simulink library "NMEA"  (R2024a)
settings: Solver=VariableStepAuto  StartTime=0.0  StopTime=10.0  RelTol=1e-3
libraries: $bdroot x44, simulink x21, simulink_extras x17, etargetslib x14
(part 2 of 4)

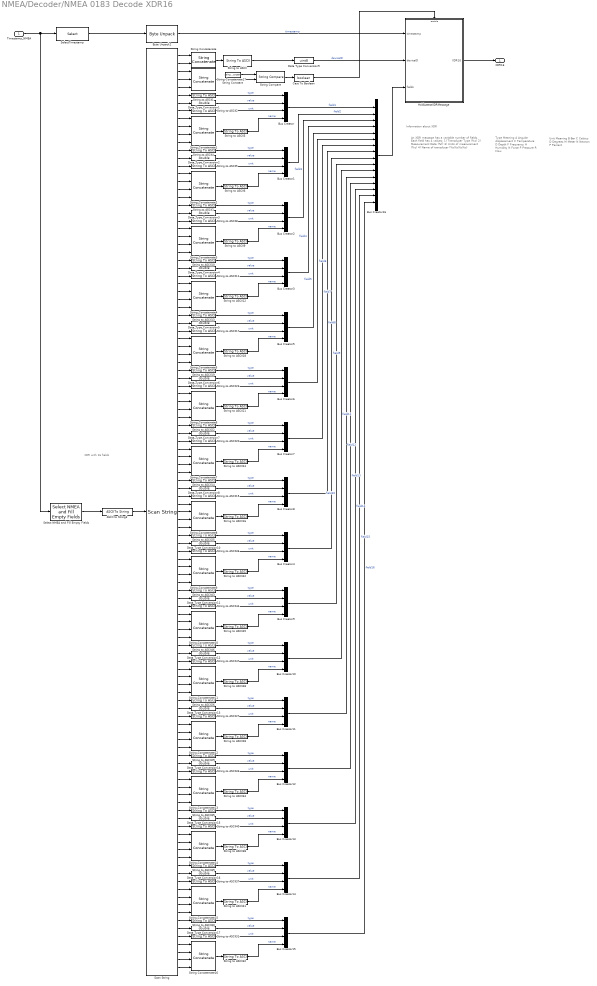
== system NMEA/Decoder/NMEA 0183 Decode XDR16 ==
  note: An XDR message has a variable number of fields.
      | Each field has 4 values:
      | 	1) Transducer Type (%c)
      | 	2) Measurement Data (%f)
      | 	3) Units of measurement (%c)
      | 	4) Name of transducer (%c%c%c%c)
  note: Type
      | Meaning
      |
      | A
      | Angular displacement
      |
      | C
      | Temperature
      |
      | D
      | Depth
      |
      | F
      | Frequency
      |
      | H
      | Humidity
      |
      | N
      | Force
      |
      | P
      | Pressure
      |
      | R
      | Flow
  note: Unit
      | Meaning
      |
      | B
      | Bar
      |
      | C
      | Celsius
      |
      | D
      | Degrees
      |
      | M
      | Meter
      |
      | N
      | Newton
      |
      | P
      | Percent
  note: Information about XDR
  note: XDR with 16 fields
  Timestamp_NMEA : Inport
  ASCII to String3 : ASCIIToString
  Bus Creator{,1..15} (16 alike) : BusCreator  Inputs=4
  Bus Creator16 : BusCreator  Inputs=16
  Byte Unpack2 : etargetslib/Byte Unpack  dimensions={1}  datatypes={'double'}  byteAlign=1
  Cast To Boolean : DataTypeConversion  OutDataTypeStr=boolean  SaturateOnIntegerOverflow=off  RndMeth=Floor
  Data Type Conversion{1..8,10..17} (16 alike) : DataTypeConversion  OutDataTypeStr=double  SaturateOnIntegerOverflow=off  RndMeth=Floor
  Data Type Conversion9 : DataTypeConversion  OutDataTypeStr=uint8  SaturateOnIntegerOverflow=off  RndMeth=Floor
  HoldLatestXDRMessage : Subsystem
  Scan String : ScanString  Format="\"$%c%c%c%c%c,%c,%lf,%c,%c%c%c%c,%c,%lf,%c,%c%c%c%c,%c,%lf,%c,%c%c%c%c,%c,%lf,%c,%c%c%c%c,%c,%lf,%c,%c%c%c%c,%c,%lf,%c,%c%c%c%c,%c,%lf,%c,%c%c%c%c,%c,%lf,%c,%c%c%c%c,%c,%lf,%c,%c%c%c%c,%c,%lf,%c,%c%c%c%c,%c,%lf,%c,%c%c%c%c,%c,%lf,%c,%c%c%c%c,%c,%lf,%c,%c%c%c%c,%c,%lf,%c,%c%c%c%c,%c,%lf,%c,%c%c%c%c,%c,%lf,%c,%c%c%c%c\""
  Select NMEA and Fill Empty Fields : $bdroot/Details/Select NMEA and Fill Empty Fields
  SelectTimestamp : Selector  IndexOptions=Index vector (dialog)  Indices=1:8  OutputSizes=1
  String Compare : StringCompare
  String Concatenate : StringConcatenate
  String Concatenate{1..16} (16 alike) : StringConcatenate  Inputs=4
  String Concatenate17 : StringConcatenate  Inputs=3
  String Constant : StringConstant  String="\"XDR\""
  String to ASCII : StringToASCII
  String to ASCII{1..2,4..5,7..8,10..11,13..15,17,19..20,22..23,25..27,29..31,33,35..37,39..40,43..44,46..47} (32 alike) : StringToASCII  OutputVectorSize=1
  String to ASCII{3,6,9,12,16,18,21,24,28,32,34,38,41..42,45,48} (16 alike) : StringToASCII  OutputVectorSize=4
  XDR16 : Outport
  wires:
  String to ASCII7/1 -> Bus Creator2/1  "type"
  Data Type Conversion3/1 -> Bus Creator2/2  "value"
  String to ASCII8/1 -> Bus Creator2/3  "unit"
  String Concatenate3/1 -> String to ASCII9/1
  String to ASCII9/1 -> Bus Creator2/4  "name"
  String to ASCII12/1 -> Bus Creator3/4  "name"
  String Concatenate4/1 -> String to ASCII12/1
  String to ASCII11/1 -> Bus Creator3/3  "unit"
  Data Type Conversion4/1 -> Bus Creator3/2  "value"
  String to ASCII10/1 -> Bus Creator3/1  "type"
  String to ASCII4/1 -> Bus Creator1/1  "type"
  Data Type Conversion2/1 -> Bus Creator1/2  "value"
  String to ASCII5/1 -> Bus Creator1/3  "unit"
  String Concatenate2/1 -> String to ASCII6/1
  String to ASCII6/1 -> Bus Creator1/4  "name"
  String to ASCII3/1 -> Bus Creator/4  "name"
  String Concatenate1/1 -> String to ASCII3/1
  String to ASCII2/1 -> Bus Creator/3  "unit"
  Data Type Conversion1/1 -> Bus Creator/2  "value"
  String to ASCII1/1 -> Bus Creator/1  "type"
  Scan String/1 -> String Concatenate/1
  Select NMEA and Fill Empty Fields/1 -> ASCII to String3/1
  SelectTimestamp/1 -> Byte Unpack2/1
  Timestamp_NMEA/1 -> Select NMEA and Fill Empty Fields/1, SelectTimestamp/1
  ASCII to String3/1 -> Scan String/1
  Scan String/2 -> String Concatenate/2
  String to ASCII13/1 -> Bus Creator5/1  "type"
  Data Type Conversion5/1 -> Bus Creator5/2  "value"
  String to ASCII17/1 -> Bus Creator5/3  "unit"
  String Concatenate5/1 -> String to ASCII18/1
  String to ASCII18/1 -> Bus Creator5/4  "name"
  String to ASCII21/1 -> Bus Creator6/4  "name"
  String Concatenate6/1 -> String to ASCII21/1
  String to ASCII23/1 -> Bus Creator6/3  "unit"
  Data Type Conversion6/1 -> Bus Creator6/2  "value"
  String to ASCII19/1 -> Bus Creator6/1  "type"
  String to ASCII14/1 -> Bus Creator8/1  "type"
  Data Type Conversion8/1 -> Bus Creator8/2  "value"
  String to ASCII15/1 -> Bus Creator8/3  "unit"
  String Concatenate8/1 -> String to ASCII16/1
  String to ASCII16/1 -> Bus Creator8/4  "name"
  String to ASCII24/1 -> Bus Creator7/4  "name"
  String Concatenate7/1 -> String to ASCII24/1
  String to ASCII20/1 -> Bus Creator7/3  "unit"
  Data Type Conversion7/1 -> Bus Creator7/2  "value"
  String to ASCII22/1 -> Bus Creator7/1  "type"
  String to ASCII/1 -> Data Type Conversion9/1
  String Concatenate/1 -> String to ASCII/1
  String to ASCII39/1 -> Bus Creator14/1  "type"
  Data Type Conversion16/1 -> Bus Creator14/2  "value"
  String to ASCII37/1 -> Bus Creator14/3  "unit"
  String Concatenate15/1 -> String to ASCII41/1
  String to ASCII41/1 -> Bus Creator14/4  "name"
  String to ASCII32/1 -> Bus Creator15/4  "name"
  String Concatenate16/1 -> String to ASCII32/1
  String to ASCII31/1 -> Bus Creator15/3  "unit"
  Data Type Conversion17/1 -> Bus Creator15/2  "value"
  String to ASCII30/1 -> Bus Creator15/1  "type"
  String to ASCII35/1 -> Bus Creator13/1  "type"
  Data Type Conversion15/1 -> Bus Creator13/2  "value"
  String to ASCII40/1 -> Bus Creator13/3  "unit"
  String Concatenate14/1 -> String to ASCII38/1
  String to ASCII38/1 -> Bus Creator13/4  "name"
  String to ASCII34/1 -> Bus Creator12/4  "name"
  String Concatenate13/1 -> String to ASCII34/1
  String to ASCII33/1 -> Bus Creator12/3  "unit"
  Data Type Conversion14/1 -> Bus Creator12/2  "value"
  String to ASCII29/1 -> Bus Creator12/1  "type"
  String to ASCII25/1 -> Bus Creator4/1  "type"
  Data Type Conversion10/1 -> Bus Creator4/2  "value"
  String to ASCII36/1 -> Bus Creator4/3  "unit"
  String Concatenate9/1 -> String to ASCII42/1
  String to ASCII42/1 -> Bus Creator4/4  "name"
  String to ASCII45/1 -> Bus Creator9/4  "name"
  String Concatenate10/1 -> String to ASCII45/1
  String to ASCII44/1 -> Bus Creator9/3  "unit"
  Data Type Conversion11/1 -> Bus Creator9/2  "value"
  String to ASCII43/1 -> Bus Creator9/1  "type"
  String to ASCII26/1 -> Bus Creator11/1  "type"
  Data Type Conversion13/1 -> Bus Creator11/2  "value"
  String to ASCII27/1 -> Bus Creator11/3  "unit"
  String Concatenate12/1 -> String to ASCII28/1
  String to ASCII28/1 -> Bus Creator11/4  "name"
  String to ASCII48/1 -> Bus Creator10/4  "name"
  String Concatenate11/1 -> String to ASCII48/1
  String to ASCII47/1 -> Bus Creator10/3  "unit"
  Data Type Conversion12/1 -> Bus Creator10/2  "value"
  String to ASCII46/1 -> Bus Creator10/1  "type"
  Scan String/3 -> String Concatenate17/1
  Scan String/4 -> String Concatenate17/2
  Scan String/5 -> String Concatenate17/3
  String Concatenate17/1 -> String Compare/2
  String Constant/1 -> String Compare/1
  String Compare/1 -> Cast To Boolean/1
  Scan String/6 -> String to ASCII1/1
  Scan String/7 -> Data Type Conversion1/1
  Scan String/8 -> String to ASCII2/1
  Scan String/9 -> String Concatenate1/1
  Scan String/10 -> String Concatenate1/2
  Scan String/11 -> String Concatenate1/3
  Scan String/12 -> String Concatenate1/4
  Scan String/13 -> String to ASCII4/1
  Scan String/14 -> Data Type Conversion2/1
  Scan String/15 -> String to ASCII5/1
  Scan String/16 -> String Concatenate2/1
  Scan String/17 -> String Concatenate2/2
  Scan String/18 -> String Concatenate2/3
  Scan String/19 -> String Concatenate2/4
  Scan String/20 -> String to ASCII7/1
  Scan String/21 -> Data Type Conversion3/1
  Scan String/22 -> String to ASCII8/1
  Scan String/23 -> String Concatenate3/1
  Scan String/24 -> String Concatenate3/2
  Scan String/25 -> String Concatenate3/3
  Scan String/26 -> String Concatenate3/4
  Scan String/27 -> String to ASCII10/1
  Scan String/28 -> Data Type Conversion4/1
  Scan String/29 -> String to ASCII11/1
  Scan String/30 -> String Concatenate4/1
  Scan String/31 -> String Concatenate4/2
  Scan String/32 -> String Concatenate4/3
  Scan String/33 -> String Concatenate4/4
  Scan String/34 -> String to ASCII13/1
  Scan String/35 -> Data Type Conversion5/1
  Scan String/36 -> String to ASCII17/1
  Scan String/37 -> String Concatenate5/1
  Scan String/38 -> String Concatenate5/2
  Scan String/39 -> String Concatenate5/3
  Scan String/40 -> String Concatenate5/4
  Scan String/41 -> String to ASCII19/1
  Scan String/42 -> Data Type Conversion6/1
  Scan String/43 -> String to ASCII23/1
  Scan String/44 -> String Concatenate6/1
  Scan String/45 -> String Concatenate6/2
  Scan String/46 -> String Concatenate6/3
  Scan String/47 -> String Concatenate6/4
  Scan String/48 -> String to ASCII22/1
  Scan String/49 -> Data Type Conversion7/1
  Scan String/50 -> String to ASCII20/1
  Scan String/51 -> String Concatenate7/1
  Scan String/52 -> String Concatenate7/2
  Scan String/53 -> String Concatenate7/3
  Scan String/54 -> String Concatenate7/4
  Scan String/55 -> String to ASCII14/1
  Scan String/56 -> Data Type Conversion8/1
  Scan String/57 -> String to ASCII15/1
  Scan String/58 -> String Concatenate8/1
  Scan String/59 -> String Concatenate8/2
  Scan String/60 -> String Concatenate8/3
  Scan String/61 -> String Concatenate8/4
  Scan String/62 -> String to ASCII25/1
  Scan String/63 -> Data Type Conversion10/1
  Scan String/64 -> String to ASCII36/1
  Scan String/65 -> String Concatenate9/1
  Scan String/66 -> String Concatenate9/2
  Scan String/67 -> String Concatenate9/3
  Scan String/68 -> String Concatenate9/4
  Scan String/69 -> String to ASCII43/1
  Scan String/70 -> Data Type Conversion11/1
  Scan String/71 -> String to ASCII44/1
  Scan String/72 -> String Concatenate10/1
  Scan String/73 -> String Concatenate10/2
  Scan String/74 -> String Concatenate10/3
  Scan String/75 -> String Concatenate10/4
  Scan String/76 -> String to ASCII46/1
  Scan String/77 -> Data Type Conversion12/1
  Scan String/78 -> String to ASCII47/1
  Scan String/79 -> String Concatenate11/1
  Scan String/80 -> String Concatenate11/2
  Scan String/81 -> String Concatenate11/3
  Scan String/82 -> String Concatenate11/4
  Scan String/83 -> String to ASCII26/1
  Scan String/84 -> Data Type Conversion13/1
  Scan String/85 -> String to ASCII27/1
  Scan String/86 -> String Concatenate12/1
  Scan String/87 -> String Concatenate12/2
  Scan String/88 -> String Concatenate12/3
  Scan String/89 -> String Concatenate12/4
  Scan String/90 -> String to ASCII29/1
  Scan String/91 -> Data Type Conversion14/1
  Scan String/92 -> String to ASCII33/1
  Scan String/93 -> String Concatenate13/1
  Scan String/94 -> String Concatenate13/2
  Scan String/95 -> String Concatenate13/3
  Scan String/96 -> String Concatenate13/4
  Scan String/97 -> String to ASCII35/1
  Scan String/98 -> Data Type Conversion15/1
  Scan String/99 -> String to ASCII40/1
  Scan String/100 -> String Concatenate14/1
  Scan String/101 -> String Concatenate14/2
  Scan String/102 -> String Concatenate14/3
  Scan String/103 -> String Concatenate14/4
  Scan String/104 -> String to ASCII39/1
  Scan String/105 -> Data Type Conversion16/1
  Scan String/106 -> String to ASCII37/1
  Scan String/107 -> String Concatenate15/1
  Scan String/108 -> String Concatenate15/2
  Scan String/109 -> String Concatenate15/3
  Scan String/110 -> String Concatenate15/4
  Scan String/111 -> String to ASCII30/1
  Scan String/112 -> Data Type Conversion17/1
  Scan String/113 -> String to ASCII31/1
  Scan String/114 -> String Concatenate16/1
  Scan String/115 -> String Concatenate16/2
  Scan String/116 -> String Concatenate16/3
  Scan String/117 -> String Concatenate16/4
  Bus Creator9/1 -> Bus Creator16/10  "field10"
  Bus Creator4/1 -> Bus Creator16/9  "field9"
  Bus Creator10/1 -> Bus Creator16/11  "field11"
  Bus Creator8/1 -> Bus Creator16/8  "field8"
  Bus Creator11/1 -> Bus Creator16/12  "field12"
  Bus Creator7/1 -> Bus Creator16/7  "field7"
  Bus Creator12/1 -> Bus Creator16/13  "field13"
  Bus Creator6/1 -> Bus Creator16/6  "field6"
  Bus Creator13/1 -> Bus Creator16/14  "field14"
  Bus Creator5/1 -> Bus Creator16/5  "field5"
  Bus Creator14/1 -> Bus Creator16/15  "field15"
  Bus Creator3/1 -> Bus Creator16/4  "field4"
  Bus Creator15/1 -> Bus Creator16/16  "field16"
  Bus Creator2/1 -> Bus Creator16/3  "field3"
  Bus Creator1/1 -> Bus Creator16/2  "field2"
  Bus Creator/1 -> Bus Creator16/1  "field1"
  Bus Creator16/1 -> HoldLatestXDRMessage/3(fields)
  Data Type Conversion9/1 -> HoldLatestXDRMessage/2(deviceID)  "deviceID"
  Byte Unpack2/1 -> HoldLatestXDRMessage/1(timestamp)  "timestamp"
  Cast To Boolean/1 -> HoldLatestXDRMessage/Enable
  HoldLatestXDRMessage/1(XDR16) -> XDR16/1

== system NMEA/Decoder/NMEA 0183 Decode ZDA ==
  Timestamp_NMEA : Inport
  ASCII to String3 : ASCIIToString
  Byte Unpack2 : etargetslib/Byte Unpack  dimensions={1}  datatypes={'double'}  byteAlign=1
  Compare To Constant : simulink/Logic and Bit Operations/Compare To Constant  relop===  const=uint8(42)  OutDataTypeStr=boolean
  DecodeMessage : Subsystem  TreatAsAtomicUnit=on
  Scan String : ScanString  Format="\"$%c%cZDA,%02u%02u%lf,%02u,%02u,%u,%02u,%02u%c\""
  Select NMEA and Fill Empty Fields : $bdroot/Details/Select NMEA and Fill Empty Fields
  SelectTimestamp : Selector  IndexOptions=Index vector (dialog)  Indices=1:8  OutputSizes=1
  String Concatenate : StringConcatenate
  String to ASCII : StringToASCII  OutputVectorSize=1
  ZDA : Outport
  wires:
  Compare To Constant/1 -> DecodeMessage/Enable
  Scan String/2 -> String Concatenate/2
  String Concatenate/1 -> DecodeMessage/2(strID)
  ASCII to String3/1 -> Scan String/1
  Timestamp_NMEA/1 -> Select NMEA and Fill Empty Fields/1, SelectTimestamp/1
  DecodeMessage/1(ZDA) -> ZDA/1
  Byte Unpack2/1 -> DecodeMessage/1(timestamp)  "timestamp"
  Scan String/11 -> String to ASCII/1
  SelectTimestamp/1 -> Byte Unpack2/1
  String to ASCII/1 -> Compare To Constant/1
  Select NMEA and Fill Empty Fields/1 -> ASCII to String3/1
  Scan String/1 -> String Concatenate/1
  Scan String/3 -> DecodeMessage/3(utcHour)
  Scan String/4 -> DecodeMessage/4(utcMinute)
  Scan String/5 -> DecodeMessage/5(utcSecond)
  Scan String/6 -> DecodeMessage/6(utcDay)
  Scan String/7 -> DecodeMessage/7(utcMonth)
  Scan String/8 -> DecodeMessage/8(utcYear)
  Scan String/9 -> DecodeMessage/9(localTimeZoneOffsetFromGMTHour)
  Scan String/10 -> DecodeMessage/10(localTimeZoneOffsetFromGMTMinute)

== system NMEA/Details/Append CR LF ==
  bytesIn : Inport  OutDataTypeStr=uint8
  lengthIn : Inport  Port=2  OutDataTypeStr=uint32  PortDimensions=1
  Assignment : Assignment  DiagnosticForDimensions=Warning  IndexOptions=Index vector (port)  Indices=1  OutputSizes=1
  Bias : Bias  Bias=int32(1)  SaturateOnIntegerOverflow=off
  Bias1 : Bias  Bias=int32(2)  SaturateOnIntegerOverflow=off
  Bias2 : Bias  Bias=uint32(2)  SaturateOnIntegerOverflow=off
  Compare To Constant : simulink/Logic and Bit Operations/Compare To Constant  relop=>  const=int32(1)  OutDataTypeStr=boolean
  Constant : Constant  Value=int32(1)
  Constant81 : Constant  Value=int32(1)
  Constant82 : Constant  Value=uint8(13)
  Constant83 : Constant  Value=uint8(10)
  Data Type Conversion : DataTypeConversion  OutDataTypeStr=int32  SaturateOnIntegerOverflow=off  RndMeth=Floor
  Mux{,1..3} (4 alike) : Mux  Inputs=2
  Selector : Selector  IndexOptions=Index vector (dialog)  Indices=1  OutputSizes=1
  Selector1 : Selector  IndexOptions=Index vector (dialog)  Indices=2  OutputSizes=1
  Sum : Sum  Inputs=|+-
  Switch : Switch  Criteria=u2 > Threshold  SaturateOnIntegerOverflow=off  InputSameDT=off
  Switch1 : Switch  Criteria=u2 > Threshold  SaturateOnIntegerOverflow=off  InputSameDT=off
  Switch2 : Switch  Criteria=u2 > Threshold  SaturateOnIntegerOverflow=off  InputSameDT=off
  Width : Width  DataType=int32
  bytesOut : Outport  OutDataTypeStr=uint8
  lengthOut : Outport  Port=2  OutDataTypeStr=uint32
  wires:
  Bias1/1 -> Mux/2
  Width/1 -> Sum/1
  Bias2/1 -> Switch2/1
  Constant/1 -> Mux1/1
  Compare To Constant/1 -> Switch2/2, Switch/2, Switch1/2
  Bias/1 -> Mux/1
  Mux3/1 -> Switch1/3
  lengthIn/1 -> Switch2/3, Bias2/1, Data Type Conversion/1
  Data Type Conversion/1 -> Bias1/1, Bias/1, Sum/2
  Mux/1 -> Switch/1
  bytesIn/1 -> Assignment/1, Selector1/1, Selector/1, Width/1
  Sum/1 -> Compare To Constant/1
  Mux2/1 -> Switch1/1
  Constant81/1 -> Mux1/2
  Constant82/1 -> Mux2/1
  Switch1/1 -> Assignment/2
  Switch/1 -> Assignment/3
  Mux1/1 -> Switch/3
  Selector/1 -> Mux3/1
  Selector1/1 -> Mux3/2
  Constant83/1 -> Mux2/2
  Assignment/1 -> bytesOut/1
  Switch2/1 -> lengthOut/1

== system NMEA/Details/Ensure Positive Angle ==
  x : Inport  OutDataTypeStr=double  Unit=rad
  Positive Angle : MATLAB Function  TreatAsAtomicUnit=on
  y : Outport  OutDataTypeStr=double  Unit=rad
  wires:
  Positive Angle/1(y) -> y/1
  x/1 -> Positive Angle/1(x)

== system NMEA/Details/Ensure Symmetrical Angle ==
  x : Inport  OutDataTypeStr=double  Unit=rad
  Symmetrical Angle : MATLAB Function  TreatAsAtomicUnit=on
  y : Outport  OutDataTypeStr=double  Unit=rad
  wires:
  x/1 -> Symmetrical Angle/1(x)
  Symmetrical Angle/1(y) -> y/1

== system NMEA/Details/NMEA Checksum Message ==
  note: Add checksum (output buffer size: 128)
  note: NMEA String including $ and *
  nmeaString : Inport
  MATLAB Function : MATLAB Function  TreatAsAtomicUnit=on
  bytes : Outport  OutDataTypeStr=uint8
  length : Outport  Port=2  OutDataTypeStr=uint32  PortDimensions=1
  wires:
  MATLAB Function/2(len) -> length/1
  MATLAB Function/1(bytes) -> bytes/1
  nmeaString/1 -> MATLAB Function/1(nmeaData)

== system NMEA/Details/NMEA Checksum Test ==
  bytes : Inport  OutDataTypeStr=uint8
  length : Inport  Port=2  OutDataTypeStr=uint32  PortDimensions=1
  MATLAB Function : MATLAB Function  TreatAsAtomicUnit=on
  isCorrect : Outport  OutDataTypeStr=boolean  PortDimensions=1
  wires:
  MATLAB Function/1(isCorrect) -> isCorrect/1
  bytes/1 -> MATLAB Function/1(bytes)
  length/1 -> MATLAB Function/2(len)

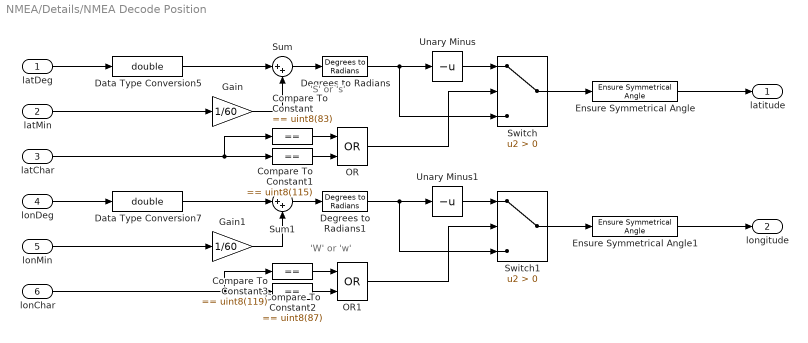
== system NMEA/Details/NMEA Decode Position ==
  note: 'S' or 's'
  note: 'W' or 'w'
  latDeg : Inport  OutDataTypeStr=uint32  Unit=deg  PortDimensions=1
  latMin : Inport  Port=2  OutDataTypeStr=double  Unit=min  PortDimensions=1
  latChar : Inport  Port=3  OutDataTypeStr=uint8  PortDimensions=1
  lonDeg : Inport  Port=4  OutDataTypeStr=uint32  Unit=deg  PortDimensions=1
  lonMin : Inport  Port=5  OutDataTypeStr=double  Unit=min  PortDimensions=1
  lonChar : Inport  Port=6  OutDataTypeStr=uint8  PortDimensions=1
  Compare To Constant : simulink/Logic and Bit Operations/Compare To Constant  relop===  const=uint8(83)  OutDataTypeStr=boolean
  Compare To Constant1 : simulink/Logic and Bit Operations/Compare To Constant  relop===  const=uint8(115)  OutDataTypeStr=boolean
  Compare To Constant2 : simulink/Logic and Bit Operations/Compare To Constant  relop===  const=uint8(87)  OutDataTypeStr=boolean
  Compare To Constant3 : simulink/Logic and Bit Operations/Compare To Constant  relop===  const=uint8(119)  OutDataTypeStr=boolean
  Data Type Conversion5 : DataTypeConversion  OutDataTypeStr=double  SaturateOnIntegerOverflow=off  RndMeth=Floor
  Data Type Conversion7 : DataTypeConversion  OutDataTypeStr=double  SaturateOnIntegerOverflow=off  RndMeth=Floor
  Degrees to Radians : simulink_extras/Transformations/Degrees to Radians
  Degrees to Radians1 : simulink_extras/Transformations/Degrees to Radians
  Ensure Symmetrical Angle : $bdroot/Details/Ensure Symmetrical Angle
  Ensure Symmetrical Angle1 : $bdroot/Details/Ensure Symmetrical Angle
  Gain : Gain  Gain=1/60
  Gain1 : Gain  Gain=1/60
  OR : Logic  Operator=OR  AllPortsSameDT=off  OutDataTypeStr=boolean
  OR1 : Logic  Operator=OR  AllPortsSameDT=off  OutDataTypeStr=boolean
  Sum : Sum  Inputs=|++
  Sum1 : Sum  Inputs=|++
  Switch : Switch  Criteria=u2 > Threshold  SaturateOnIntegerOverflow=off  InputSameDT=off
  Switch1 : Switch  Criteria=u2 > Threshold  SaturateOnIntegerOverflow=off  InputSameDT=off
  Unary Minus : UnaryMinus
  Unary Minus1 : UnaryMinus
  latitude : Outport  OutDataTypeStr=double  Unit=rad  PortDimensions=1
  longitude : Outport  Port=2  OutDataTypeStr=double  Unit=rad  PortDimensions=1
  wires:
  Data Type Conversion5/1 -> Sum/1
  Switch1/1 -> Ensure Symmetrical Angle1/1
  latDeg/1 -> Data Type Conversion5/1
  lonChar/1 -> Compare To Constant3/1, Compare To Constant2/1
  latMin/1 -> Gain/1
  Data Type Conversion7/1 -> Sum1/1
  Gain/1 -> Sum/2
  Compare To Constant/1 -> OR/1
  Unary Minus1/1 -> Switch1/1
  Sum/1 -> Degrees to Radians/1
  lonMin/1 -> Gain1/1
  Compare To Constant3/1 -> OR1/2
  latChar/1 -> Compare To Constant/1, Compare To Constant1/1
  OR/1 -> Switch/2
  Compare To Constant1/1 -> OR/2
  Unary Minus/1 -> Switch/1
  OR1/1 -> Switch1/2
  Gain1/1 -> Sum1/2
  Degrees to Radians/1 -> Switch/3, Unary Minus/1
  Sum1/1 -> Degrees to Radians1/1
  Degrees to Radians1/1 -> Unary Minus1/1, Switch1/3
  lonDeg/1 -> Data Type Conversion7/1
  Switch/1 -> Ensure Symmetrical Angle/1
  Compare To Constant2/1 -> OR1/1
  Ensure Symmetrical Angle/1 -> latitude/1
  Ensure Symmetrical Angle1/1 -> longitude/1

== system NMEA/Details/NMEA Encode Position ==
  lat : Inport  OutDataTypeStr=double  Unit=rad  PortDimensions=1
  lon : Inport  Port=2  OutDataTypeStr=double  Unit=rad  PortDimensions=1
  EncodePosition : MATLAB Function  TreatAsAtomicUnit=on
  latDeg : Outport  OutDataTypeStr=uint32  Unit=deg  PortDimensions=1
  latMin : Outport  Port=2  OutDataTypeStr=double  Unit=min  PortDimensions=1
  latChar : Outport  Port=3  OutDataTypeStr=uint8  PortDimensions=1
  lonDeg : Outport  Port=4  OutDataTypeStr=uint32  Unit=deg  PortDimensions=1
  lonMin : Outport  Port=5  OutDataTypeStr=double  Unit=min  PortDimensions=1
  lonChar : Outport  Port=6  OutDataTypeStr=uint8  PortDimensions=1
  wires:
  EncodePosition/2(latMin) -> latMin/1
  lat/1 -> EncodePosition/1(lat)
  lon/1 -> EncodePosition/2(lon)
  EncodePosition/3(latChar) -> latChar/1
  EncodePosition/4(lonDeg) -> lonDeg/1
  EncodePosition/1(latDeg) -> latDeg/1
  EncodePosition/6(lonChar) -> lonChar/1
  EncodePosition/5(lonMin) -> lonMin/1

== system NMEA/Details/NMEA Fill Empty Fields ==
  bytesIn : Inport  OutDataTypeStr=uint8
  lengthIn : Inport  Port=2  OutDataTypeStr=uint32  PortDimensions=1
  MATLAB Function : MATLAB Function  TreatAsAtomicUnit=on
  bytesOut : Outport  OutDataTypeStr=uint8
  lengthOut : Outport  Port=2  OutDataTypeStr=uint32  PortDimensions=1
  wires:
  MATLAB Function/1(bytesOut) -> bytesOut/1
  lengthIn/1 -> MATLAB Function/2(lengthIn)
  MATLAB Function/2(lengthOut) -> lengthOut/1
  bytesIn/1 -> MATLAB Function/1(bytesIn)

== system NMEA/Details/NMEA XDR16 Get Value Of Transducer ==
  note: Unit
      | Meaning
      |
      | B
      | Bar
      |
      | C
      | Celsius
      |
      | D
      | Degrees
      |
      | M
      | Meter
      |
      | N
      | Newton
      |
      | P
      | Percent
  note: Type
      | Meaning
      |
      | A
      | Angular displacement
      |
      | C
      | Temperature
      |
      | D
      | Depth
      |
      | F
      | Frequency
      |
      | H
      | Humidity
      |
      | N
      | Force
      |
      | P
      | Pressure
      |
      | R
      | Flow
  note: Information about XDR
  note: An XDR message has a variable number of fields.
      | Each field has 4 values:
      | 	1) Transducer Type (%c)
      | 	2) Measurement Data (%f)
      | 	3) Units of measurement (%c)
      | 	4) Name of transducer (%c%c%c%c)
  transducerName : Inport  OutDataTypeStr=uint8  PortDimensions=4
  XDR16 : Inport  Port=2
  Bus Selector1 : BusSelector  OutputSignals=types,values,units,names
  MATLAB Function : MATLAB Function  TreatAsAtomicUnit=on
  found : Outport  OutDataTypeStr=boolean  PortDimensions=1
  value : Outport  Port=2  OutDataTypeStr=double  PortDimensions=1
  wires:
  MATLAB Function/1(value) -> value/1
  Bus Selector1/4 -> MATLAB Function/5(namesXDR)  "<names>"
  XDR16/1 -> Bus Selector1/1
  Bus Selector1/1 -> MATLAB Function/2(typesXDR)  "<types>"
  Bus Selector1/2 -> MATLAB Function/3(valuesXDR)  "<values>"
  transducerName/1 -> MATLAB Function/1(transducerName)
  Bus Selector1/3 -> MATLAB Function/4(unitsXDR)  "<units>"
  MATLAB Function/2(found) -> found/1

== system NMEA/Details/Select NMEA and Fill Empty Fields ==
  Timestamp_NMEA : Inport
  SelectMessageAndFillEmptyFields : MATLAB Function  TreatAsAtomicUnit=on
  ASCII : Outport
  wires:
  Timestamp_NMEA/1 -> SelectMessageAndFillEmptyFields/1(u)
  SelectMessageAndFillEmptyFields/1(y) -> ASCII/1

== system NMEA/Encoder/NMEA 0183 Encode ALR ==
  note: Add checksum (output buffer size: 128)
  note: NMEA String including $ and *
  deviceID : Inport  OutDataTypeStr=uint8  PortDimensions=2
  utcHour : Inport  Port=2  OutDataTypeStr=uint32  PortDimensions=1
  utcMinute : Inport  Port=3  OutDataTypeStr=uint32  PortDimensions=1
  utcSecond : Inport  Port=4  OutDataTypeStr=double  Unit=s  PortDimensions=1
  alarmID1 : Inport  Port=5  OutDataTypeStr=uint32  PortDimensions=1
  alarmID2 : Inport  Port=6  OutDataTypeStr=uint32  PortDimensions=1
  alarmID3 : Inport  Port=7  OutDataTypeStr=uint32  PortDimensions=1
  alarmCondition : Inport  Port=8  OutDataTypeStr=uint8  PortDimensions=1
  alarmAcknowledge : Inport  Port=9  OutDataTypeStr=uint8  PortDimensions=1
  ASCII to String : ASCIIToString
  ASCII to String1 : ASCIIToString
  ASCII to String2 : ASCIIToString
  Compose String : ComposeString  Format="\"$%sALR,%02u%02u%05.2f,%u%u%u,%s,%s,*\""
  NMEA Checksum Message : $bdroot/Details/NMEA Checksum Message
  Saturation : Saturate  UpperLimit=uint32(9)  LowerLimit=uint32(0)
  Saturation1 : Saturate  UpperLimit=uint32(9)  LowerLimit=uint32(0)
  Saturation2 : Saturate  UpperLimit=uint32(9)  LowerLimit=uint32(0)
  bytes : Outport  OutDataTypeStr=uint8
  length : Outport  Port=2  OutDataTypeStr=uint32  PortDimensions=1
  wires:
  NMEA Checksum Message/1 -> bytes/1
  NMEA Checksum Message/2 -> length/1
  deviceID/1 -> ASCII to String/1
  ASCII to String/1 -> Compose String/1
  Compose String/1 -> NMEA Checksum Message/1
  utcHour/1 -> Compose String/2
  utcMinute/1 -> Compose String/3
  utcSecond/1 -> Compose String/4
  alarmID1/1 -> Saturation/1
  alarmID2/1 -> Saturation1/1
  alarmID3/1 -> Saturation2/1
  alarmCondition/1 -> ASCII to String1/1
  ASCII to String1/1 -> Compose String/8
  alarmAcknowledge/1 -> ASCII to String2/1
  ASCII to String2/1 -> Compose String/9
  Saturation/1 -> Compose String/5
  Saturation1/1 -> Compose String/6
  Saturation2/1 -> Compose String/7

== system NMEA/Encoder/NMEA 0183 Encode DBT ==
  note: Add checksum (output buffer size: 128)
  note: NMEA String including $ and *
  deviceID : Inport  OutDataTypeStr=uint8  PortDimensions=2
  depth1 : Inport  Port=2  OutDataTypeStr=double  Unit=m  PortDimensions=1
  depth2 : Inport  Port=3  OutDataTypeStr=double  Unit=m  PortDimensions=1
  depth3 : Inport  Port=4  OutDataTypeStr=double  Unit=m  PortDimensions=1
  ASCII to String : ASCIIToString
  Compose String : ComposeString  Format="\"$%sDBT,%.1f,f,%.1f,M,%.1f,F*\""
  Gain : Gain  Gain=3.28083333333333
  Gain2 : Gain  Gain=1/1.8288
  NMEA Checksum Message : $bdroot/Details/NMEA Checksum Message
  bytes : Outport  OutDataTypeStr=uint8
  length : Outport  Port=2  OutDataTypeStr=uint32  PortDimensions=1
  wires:
  NMEA Checksum Message/1 -> bytes/1
  NMEA Checksum Message/2 -> length/1
  deviceID/1 -> ASCII to String/1
  ASCII to String/1 -> Compose String/1
  depth3/1 -> Gain2/1
  depth1/1 -> Gain/1
  Gain/1 -> Compose String/2
  Gain2/1 -> Compose String/4  "depth3"
  depth2/1 -> Compose String/3
  Compose String/1 -> NMEA Checksum Message/1

== system NMEA/Encoder/NMEA 0183 Encode GGA ==
  note: NMEA String including $ and *
  note: Add checksum (output buffer size: 128)
  deviceID : Inport  OutDataTypeStr=uint8  PortDimensions=2
  utcHour : Inport  Port=2  OutDataTypeStr=uint32  PortDimensions=1
  utcMinute : Inport  Port=3  OutDataTypeStr=uint32  PortDimensions=1
  utcSecond : Inport  Port=4  OutDataTypeStr=double  Unit=s  PortDimensions=1
  latitude : Inport  Port=5  OutDataTypeStr=double  Unit=rad  PortDimensions=1
  longitude : Inport  Port=6  OutDataTypeStr=double  Unit=rad  PortDimensions=1
  gpsQuality : Inport  Port=7  OutDataTypeStr=uint32  PortDimensions=1
  numSat : Inport  Port=8  OutDataTypeStr=uint32  PortDimensions=1
  hdop : Inport  Port=9  OutDataTypeStr=double  PortDimensions=1
  antennaHeightMSL : Inport  Port=10  OutDataTypeStr=double  Unit=m  PortDimensions=1
  geoidSeparation : Inport  Port=11  OutDataTypeStr=double  Unit=m  PortDimensions=1
  ageOfDGPS : Inport  Port=12  OutDataTypeStr=double  Unit=s  PortDimensions=1
  dgpsReferenceStation : Inport  Port=13  OutDataTypeStr=uint32  PortDimensions=1
  ASCII to String : ASCIIToString
  ASCII to String1 : ASCIIToString
  ASCII to String2 : ASCIIToString
  Compose String : ComposeString  Format="\"$%sGGA,%02u%02u%05.2f,%02u%010.7f,%s,%03u%010.7f,%s,%u,%u,%.3f,%.3f,M,%.3f,M,%.1f,%04u*\""
  NMEA Checksum Message : $bdroot/Details/NMEA Checksum Message
  NMEA Encode Position : $bdroot/Details/NMEA Encode Position
  Saturation : Saturate  UpperLimit=1023  LowerLimit=0
  bytes : Outport  OutDataTypeStr=uint8
  length : Outport  Port=2  OutDataTypeStr=uint32  PortDimensions=1
  wires:
  ASCII to String/1 -> Compose String/1
  hdop/1 -> Compose String/13
  utcHour/1 -> Compose String/2
  utcSecond/1 -> Compose String/4
  dgpsReferenceStation/1 -> Saturation/1
  Compose String/1 -> NMEA Checksum Message/1
  gpsQuality/1 -> Compose String/11
  utcMinute/1 -> Compose String/3
  numSat/1 -> Compose String/12
  deviceID/1 -> ASCII to String/1
  latitude/1 -> NMEA Encode Position/1
  longitude/1 -> NMEA Encode Position/2
  NMEA Encode Position/1 -> Compose String/5
  NMEA Encode Position/2 -> Compose String/6
  NMEA Encode Position/3 -> ASCII to String1/1
  NMEA Encode Position/4 -> Compose String/8
  NMEA Encode Position/5 -> Compose String/9
  NMEA Encode Position/6 -> ASCII to String2/1
  ASCII to String1/1 -> Compose String/7
  ASCII to String2/1 -> Compose String/10
  NMEA Checksum Message/1 -> bytes/1
  NMEA Checksum Message/2 -> length/1
  antennaHeightMSL/1 -> Compose String/14
  geoidSeparation/1 -> Compose String/15
  ageOfDGPS/1 -> Compose String/16
  Saturation/1 -> Compose String/17

== system NMEA/Encoder/NMEA 0183 Encode HDT ==
  note: NMEA String including $ and *
  note: Add checksum (output buffer size: 128)
  deviceID : Inport  OutDataTypeStr=uint8  PortDimensions=2
  trueHeading : Inport  Port=2  OutDataTypeStr=double  Unit=rad  PortDimensions=1
  ASCII to String : ASCIIToString
  Compose String : ComposeString  Format="\"$%sHDT,%.2f,T*\""
  NMEA Checksum Message : $bdroot/Details/NMEA Checksum Message
  Radians to Degrees : simulink_extras/Transformations/Radians to Degrees
  bytes : Outport  OutDataTypeStr=uint8
  length : Outport  Port=2  OutDataTypeStr=uint32  PortDimensions=1
  wires:
  NMEA Checksum Message/1 -> bytes/1
  NMEA Checksum Message/2 -> length/1
  ASCII to String/1 -> Compose String/1
  Compose String/1 -> NMEA Checksum Message/1
  deviceID/1 -> ASCII to String/1
  trueHeading/1 -> Radians to Degrees/1
  Radians to Degrees/1 -> Compose String/2

== system NMEA/Encoder/NMEA 0183 Encode MWV ==
  note: NMEA String including $ and *
  note: Add checksum (output buffer size: 128)
  deviceID : Inport  OutDataTypeStr=uint8  PortDimensions=2
  windAngle : Inport  Port=2  OutDataTypeStr=double  Unit=rad  PortDimensions=1
  windAngleReference : Inport  Port=3  OutDataTypeStr=uint8  PortDimensions=1
  windSpeed : Inport  Port=4  OutDataTypeStr=double  Unit=m/s  PortDimensions=1
  status : Inport  Port=5  OutDataTypeStr=uint8  PortDimensions=1
  ASCII to String : ASCIIToString
  ASCII to String1 : ASCIIToString
  ASCII to String2 : ASCIIToString
  Compose String : ComposeString  Format="\"$%sMWV,%05.1f,%s,%.1f,M,%s*\""
  Ensure Positive Angle : $bdroot/Details/Ensure Positive Angle
  NMEA Checksum Message : $bdroot/Details/NMEA Checksum Message
  Radians to Degrees : simulink_extras/Transformations/Radians to Degrees
  bytes : Outport  OutDataTypeStr=uint8
  length : Outport  Port=2  OutDataTypeStr=uint32  PortDimensions=1
  wires:
  NMEA Checksum Message/1 -> bytes/1
  NMEA Checksum Message/2 -> length/1
  Compose String/1 -> NMEA Checksum Message/1
  ASCII to String/1 -> Compose String/1
  deviceID/1 -> ASCII to String/1
  windAngle/1 -> Ensure Positive Angle/1
  Ensure Positive Angle/1 -> Radians to Degrees/1
  Radians to Degrees/1 -> Compose String/2
  ASCII to String1/1 -> Compose String/3
  windAngleReference/1 -> ASCII to String1/1
  windSpeed/1 -> Compose String/4
  status/1 -> ASCII to String2/1
  ASCII to String2/1 -> Compose String/5

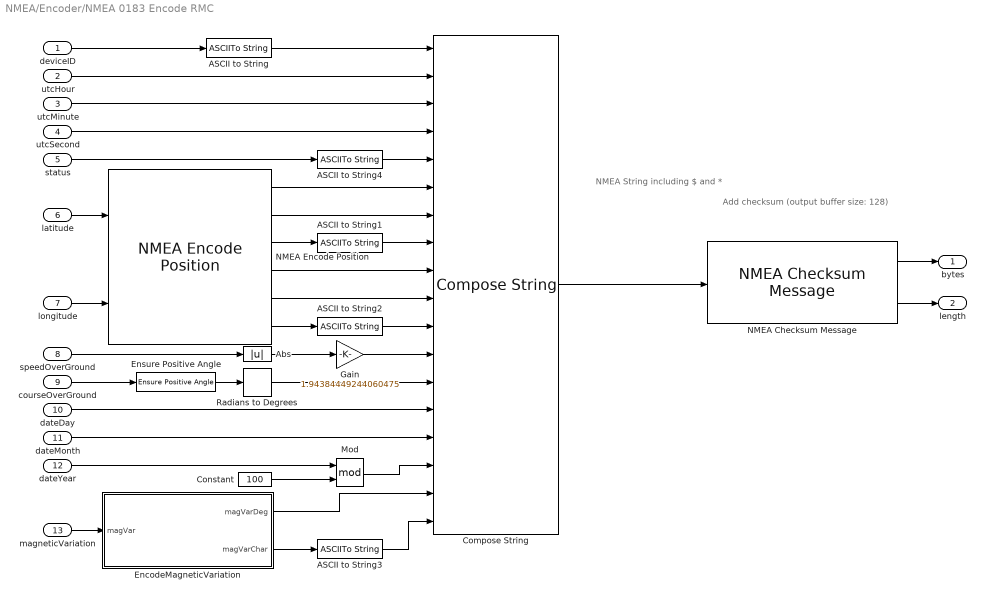
== system NMEA/Encoder/NMEA 0183 Encode RMC ==
  note: Add checksum (output buffer size: 128)
  note: NMEA String including $ and *
  deviceID : Inport  OutDataTypeStr=uint8  PortDimensions=2
  utcHour : Inport  Port=2  OutDataTypeStr=uint32  PortDimensions=1
  utcMinute : Inport  Port=3  OutDataTypeStr=uint32  PortDimensions=1
  utcSecond : Inport  Port=4  OutDataTypeStr=double  Unit=s  PortDimensions=1
  status : Inport  Port=5  OutDataTypeStr=uint8  PortDimensions=1
  latitude : Inport  Port=6  OutDataTypeStr=double  Unit=rad  PortDimensions=1
  longitude : Inport  Port=7  OutDataTypeStr=double  Unit=rad  PortDimensions=1
  speedOverGround : Inport  Port=8  OutDataTypeStr=double  Unit=m/s  PortDimensions=1
  courseOverGround : Inport  Port=9  OutDataTypeStr=double  Unit=rad  PortDimensions=1
  dateDay : Inport  Port=10  OutDataTypeStr=uint32  PortDimensions=1
  dateMonth : Inport  Port=11  OutDataTypeStr=uint32  PortDimensions=1
  dateYear : Inport  Port=12  OutDataTypeStr=uint32  PortDimensions=1
  magneticVariation : Inport  Port=13  OutDataTypeStr=double  Unit=rad  PortDimensions=1
  ASCII to String{,1..4} (5 alike) : ASCIIToString
  Abs : Abs  SaturateOnIntegerOverflow=off
  Compose String : ComposeString  Format="\"$%sRMC,%02u%02u%05.2f,%s,%02u%010.7f,%s,%03u%010.7f,%s,%05.1f,%05.1f,%02u%02u%02u,%05.1f,%s*\""
  Constant : Constant  Value=100  OutDataTypeStr=uint32
  EncodeMagneticVariation : MATLAB Function  TreatAsAtomicUnit=on
  Ensure Positive Angle : $bdroot/Details/Ensure Positive Angle
  Gain : Gain  Gain=1.94384449244060475
  Mod : Math  Operator=mod
  NMEA Checksum Message : $bdroot/Details/NMEA Checksum Message
  NMEA Encode Position : $bdroot/Details/NMEA Encode Position
  Radians to Degrees : simulink_extras/Transformations/Radians to Degrees
  bytes : Outport  OutDataTypeStr=uint8
  length : Outport  Port=2  OutDataTypeStr=uint32  PortDimensions=1
  wires:
  NMEA Checksum Message/2 -> length/1
  NMEA Checksum Message/1 -> bytes/1
  NMEA Encode Position/6 -> ASCII to String2/1
  NMEA Encode Position/3 -> ASCII to String1/1
  longitude/1 -> NMEA Encode Position/2
  latitude/1 -> NMEA Encode Position/1
  deviceID/1 -> ASCII to String/1
  utcMinute/1 -> Compose String/3
  Compose String/1 -> NMEA Checksum Message/1
  utcSecond/1 -> Compose String/4
  utcHour/1 -> Compose String/2
  ASCII to String/1 -> Compose String/1
  status/1 -> ASCII to String4/1
  NMEA Encode Position/1 -> Compose String/6
  NMEA Encode Position/2 -> Compose String/7
  ASCII to String1/1 -> Compose String/8
  NMEA Encode Position/4 -> Compose String/9
  NMEA Encode Position/5 -> Compose String/10
  ASCII to String2/1 -> Compose String/11
  Gain/1 -> Compose String/12
  speedOverGround/1 -> Abs/1
  Ensure Positive Angle/1 -> Radians to Degrees/1
  courseOverGround/1 -> Ensure Positive Angle/1
  Radians to Degrees/1 -> Compose String/13
  dateDay/1 -> Compose String/14
  dateMonth/1 -> Compose String/15
  dateYear/1 -> Mod/1
  Constant/1 -> Mod/2
  Mod/1 -> Compose String/16
  magneticVariation/1 -> EncodeMagneticVariation/1(magVar)
  EncodeMagneticVariation/2(magVarChar) -> ASCII to String3/1
  ASCII to String3/1 -> Compose String/18
  EncodeMagneticVariation/1(magVarDeg) -> Compose String/17
  ASCII to String4/1 -> Compose String/5
  Abs/1 -> Gain/1

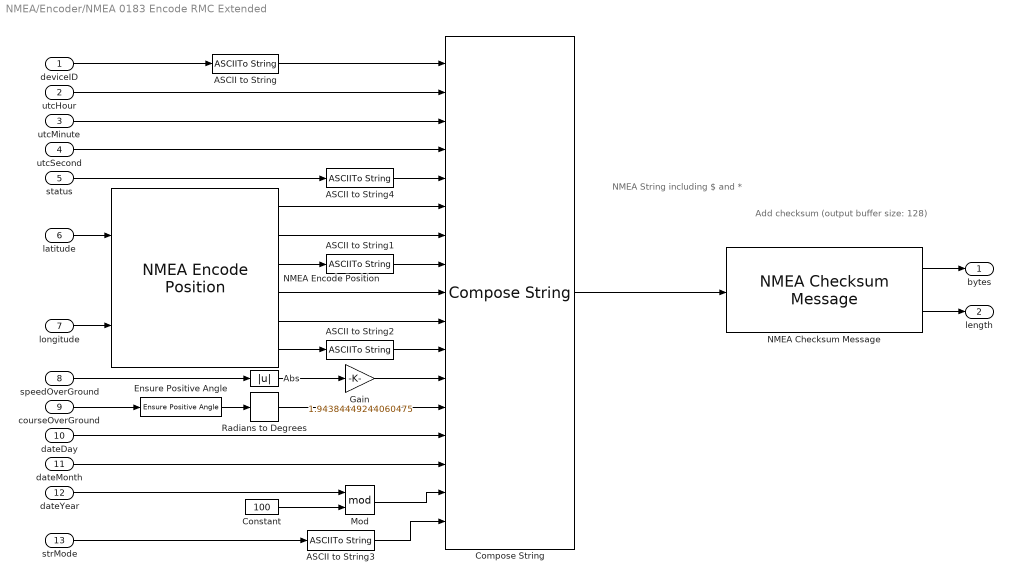
== system NMEA/Encoder/NMEA 0183 Encode RMC Extended ==
  note: NMEA String including $ and *
  note: Add checksum (output buffer size: 128)
  deviceID : Inport  OutDataTypeStr=uint8  PortDimensions=2
  utcHour : Inport  Port=2  OutDataTypeStr=uint32  PortDimensions=1
  utcMinute : Inport  Port=3  OutDataTypeStr=uint32  PortDimensions=1
  utcSecond : Inport  Port=4  OutDataTypeStr=double  Unit=s  PortDimensions=1
  status : Inport  Port=5  OutDataTypeStr=uint8  PortDimensions=1
  latitude : Inport  Port=6  OutDataTypeStr=double  Unit=rad  PortDimensions=1
  longitude : Inport  Port=7  OutDataTypeStr=double  Unit=rad  PortDimensions=1
  speedOverGround : Inport  Port=8  OutDataTypeStr=double  Unit=m/s  PortDimensions=1
  courseOverGround : Inport  Port=9  OutDataTypeStr=double  Unit=rad  PortDimensions=1
  dateDay : Inport  Port=10  OutDataTypeStr=uint32  PortDimensions=1
  dateMonth : Inport  Port=11  OutDataTypeStr=uint32  PortDimensions=1
  dateYear : Inport  Port=12  OutDataTypeStr=uint32  PortDimensions=1
  strMode : Inport  Port=13  OutDataTypeStr=uint8  PortDimensions=1
  ASCII to String{,1..4} (5 alike) : ASCIIToString
  Abs : Abs  SaturateOnIntegerOverflow=off
  Compose String : ComposeString  Format="\"$%sRMC,%02u%02u%05.2f,%s,%02u%010.7f,%s,%03u%010.7f,%s,%05.1f,%05.1f,%02u%02u%02u,0,0,%s,V*\""
  Constant : Constant  Value=100  OutDataTypeStr=uint32
  Ensure Positive Angle : $bdroot/Details/Ensure Positive Angle
  Gain : Gain  Gain=1.94384449244060475
  Mod : Math  Operator=mod
  NMEA Checksum Message : $bdroot/Details/NMEA Checksum Message
  NMEA Encode Position : $bdroot/Details/NMEA Encode Position
  Radians to Degrees : simulink_extras/Transformations/Radians to Degrees
  bytes : Outport  OutDataTypeStr=uint8
  length : Outport  Port=2  OutDataTypeStr=uint32  PortDimensions=1
  wires:
  NMEA Checksum Message/2 -> length/1
  NMEA Checksum Message/1 -> bytes/1
  ASCII to String3/1 -> Compose String/17
  Abs/1 -> Gain/1
  ASCII to String4/1 -> Compose String/5
  strMode/1 -> ASCII to String3/1
  Mod/1 -> Compose String/16
  Constant/1 -> Mod/2
  dateYear/1 -> Mod/1
  dateMonth/1 -> Compose String/15
  dateDay/1 -> Compose String/14
  Radians to Degrees/1 -> Compose String/13
  courseOverGround/1 -> Ensure Positive Angle/1
  Ensure Positive Angle/1 -> Radians to Degrees/1
  speedOverGround/1 -> Abs/1
  Gain/1 -> Compose String/12
  ASCII to String2/1 -> Compose String/11
  NMEA Encode Position/5 -> Compose String/10
  NMEA Encode Position/4 -> Compose String/9
  ASCII to String1/1 -> Compose String/8
  NMEA Encode Position/2 -> Compose String/7
  NMEA Encode Position/1 -> Compose String/6
  status/1 -> ASCII to String4/1
  ASCII to String/1 -> Compose String/1
  utcHour/1 -> Compose String/2
  utcSecond/1 -> Compose String/4
  Compose String/1 -> NMEA Checksum Message/1
  utcMinute/1 -> Compose String/3
  deviceID/1 -> ASCII to String/1
  latitude/1 -> NMEA Encode Position/1
  longitude/1 -> NMEA Encode Position/2
  NMEA Encode Position/3 -> ASCII to String1/1
  NMEA Encode Position/6 -> ASCII to String2/1

== system NMEA/Encoder/NMEA 0183 Encode ROT ==
  note: Add checksum (output buffer size: 128)
  note: NMEA String including $ and *
  deviceID : Inport  OutDataTypeStr=uint8  PortDimensions=2
  rateOfTurn : Inport  Port=2  OutDataTypeStr=double  Unit=rad/s  PortDimensions=1
  status : Inport  Port=3  OutDataTypeStr=uint8  PortDimensions=1
  ASCII to String : ASCIIToString
  ASCII to String1 : ASCIIToString
  Compose String : ComposeString  Format="\"$%sROT,%.1f,%s*\""
  Gain : Gain  Gain=60
  NMEA Checksum Message : $bdroot/Details/NMEA Checksum Message
  Radians to Degrees : simulink_extras/Transformations/Radians to Degrees
  bytes : Outport  OutDataTypeStr=uint8
  length : Outport  Port=2  OutDataTypeStr=uint32  PortDimensions=1
  wires:
  NMEA Checksum Message/1 -> bytes/1
  NMEA Checksum Message/2 -> length/1
  Radians to Degrees/1 -> Gain/1
  rateOfTurn/1 -> Radians to Degrees/1
  deviceID/1 -> ASCII to String/1
  Compose String/1 -> NMEA Checksum Message/1
  ASCII to String/1 -> Compose String/1
  ASCII to String1/1 -> Compose String/3
  status/1 -> ASCII to String1/1
  Gain/1 -> Compose String/2

== system NMEA/Encoder/NMEA 0183 Encode VBW ==
  note: Add checksum (output buffer size: 128)
  note: NMEA String including $ and *
  deviceID : Inport  OutDataTypeStr=uint8  PortDimensions=2
  waterSpeedX : Inport  Port=2  OutDataTypeStr=double  Unit=m/s  PortDimensions=1
  waterSpeedY : Inport  Port=3  OutDataTypeStr=double  Unit=m/s  PortDimensions=1
  waterSpeedStatus : Inport  Port=4  OutDataTypeStr=uint8  PortDimensions=1
  groundSpeedX : Inport  Port=5  OutDataTypeStr=double  Unit=m/s  PortDimensions=1
  groundSpeedY : Inport  Port=6  OutDataTypeStr=double  Unit=m/s  PortDimensions=1
  groundSpeedStatus : Inport  Port=7  OutDataTypeStr=uint8  PortDimensions=1
  ASCII to String : ASCIIToString
  ASCII to String1 : ASCIIToString
  ASCII to String2 : ASCIIToString
  Compose String : ComposeString  Format="\"$%sVBW,%.3f,%.3f,%s,%.3f,%.3f,%s*\""
  Gain{,1..3} (4 alike) : Gain  Gain=1.94384449244060475
  NMEA Checksum Message : $bdroot/Details/NMEA Checksum Message
  bytes : Outport  OutDataTypeStr=uint8
  length : Outport  Port=2  OutDataTypeStr=uint32  PortDimensions=1
  wires:
  NMEA Checksum Message/2 -> length/1
  NMEA Checksum Message/1 -> bytes/1
  deviceID/1 -> ASCII to String/1
  Compose String/1 -> NMEA Checksum Message/1
  ASCII to String/1 -> Compose String/1
  waterSpeedX/1 -> Gain/1
  waterSpeedY/1 -> Gain1/1
  Gain/1 -> Compose String/2
  Gain1/1 -> Compose String/3
  Gain2/1 -> Compose String/5
  Gain3/1 -> Compose String/6
  groundSpeedX/1 -> Gain2/1
  groundSpeedY/1 -> Gain3/1
  waterSpeedStatus/1 -> ASCII to String1/1
  ASCII to String1/1 -> Compose String/4
  ASCII to String2/1 -> Compose String/7
  groundSpeedStatus/1 -> ASCII to String2/1

== system NMEA/Encoder/NMEA 0183 Encode VTG ==
  note: NMEA String including $ and *
  note: Add checksum (output buffer size: 128)
  deviceID : Inport  OutDataTypeStr=uint8  PortDimensions=2
  trackMadeGoodTrue : Inport  Port=2  OutDataTypeStr=double  Unit=rad  PortDimensions=1
  trackMadeGoodMagnetic : Inport  Port=3  OutDataTypeStr=double  Unit=rad  PortDimensions=1
  speedOverGround1 : Inport  Port=4  OutDataTypeStr=double  Unit=m/s  PortDimensions=1
  speedOverGround2 : Inport  Port=5  OutDataTypeStr=double  Unit=m/s  PortDimensions=1
  ASCII to String : ASCIIToString
  Abs : Abs  SaturateOnIntegerOverflow=off
  Abs1 : Abs  SaturateOnIntegerOverflow=off
  Compose String : ComposeString  Format="\"$%sVTG,%05.1f,T,%05.1f,M,%05.1f,N,%05.1f,K*\""
  Ensure Positive Angle : $bdroot/Details/Ensure Positive Angle
  Ensure Positive Angle1 : $bdroot/Details/Ensure Positive Angle
  MPS2KPH : Gain  Gain=3.6
  MPS2Knots : Gain  Gain=1.94384449244060475
  NMEA Checksum Message : $bdroot/Details/NMEA Checksum Message
  Radians to Degrees1 : simulink_extras/Transformations/Radians to Degrees
  Radians to Degrees2 : simulink_extras/Transformations/Radians to Degrees
  bytes : Outport  OutDataTypeStr=uint8
  length : Outport  Port=2  OutDataTypeStr=uint32  PortDimensions=1
  wires:
  NMEA Checksum Message/2 -> length/1
  NMEA Checksum Message/1 -> bytes/1
  ASCII to String/1 -> Compose String/1
  Compose String/1 -> NMEA Checksum Message/1
  deviceID/1 -> ASCII to String/1
  Ensure Positive Angle/1 -> Radians to Degrees1/1
  trackMadeGoodTrue/1 -> Ensure Positive Angle/1
  Ensure Positive Angle1/1 -> Radians to Degrees2/1
  trackMadeGoodMagnetic/1 -> Ensure Positive Angle1/1
  speedOverGround1/1 -> Abs/1
  speedOverGround2/1 -> Abs1/1
  Abs/1 -> MPS2Knots/1
  Abs1/1 -> MPS2KPH/1
  MPS2Knots/1 -> Compose String/4
  MPS2KPH/1 -> Compose String/5
  Radians to Degrees2/1 -> Compose String/3
  Radians to Degrees1/1 -> Compose String/2

== system NMEA/Encoder/NMEA 0183 Encode ZDA ==
  note: Add checksum (output buffer size: 128)
  note: NMEA String including $ and *
  deviceID : Inport  OutDataTypeStr=uint8  PortDimensions=2
  utcHour : Inport  Port=2  OutDataTypeStr=uint32  PortDimensions=1
  utcMinute : Inport  Port=3  OutDataTypeStr=uint32  PortDimensions=1
  utcSecond : Inport  Port=4  OutDataTypeStr=double  Unit=s  PortDimensions=1
  utcDay : Inport  Port=5  OutDataTypeStr=uint32  PortDimensions=1
  utcMonth : Inport  Port=6  OutDataTypeStr=uint32  PortDimensions=1
  utcYear : Inport  Port=7  OutDataTypeStr=uint32  PortDimensions=1
  localTimeZoneOffsetFromGMTHour : Inport  Port=8  OutDataTypeStr=uint32  PortDimensions=1
  localTimeZoneOffsetFromGMTMinute : Inport  Port=9  OutDataTypeStr=uint32  PortDimensions=1
  ASCII to String : ASCIIToString
  Compose String : ComposeString  Format="\"$%sZDA,%02u%02u%05.2f,%02u,%02u,%u,%02u,%02u*\""
  NMEA Checksum Message : $bdroot/Details/NMEA Checksum Message
  bytes : Outport  OutDataTypeStr=uint8
  length : Outport  Port=2  OutDataTypeStr=uint32  PortDimensions=1
  wires:
  NMEA Checksum Message/2 -> length/1
  NMEA Checksum Message/1 -> bytes/1
  deviceID/1 -> ASCII to String/1
  utcMinute/1 -> Compose String/3
  Compose String/1 -> NMEA Checksum Message/1
  utcSecond/1 -> Compose String/4
  utcHour/1 -> Compose String/2
  ASCII to String/1 -> Compose String/1
  utcDay/1 -> Compose String/5
  utcMonth/1 -> Compose String/6
  utcYear/1 -> Compose String/7
  localTimeZoneOffsetFromGMTHour/1 -> Compose String/8
  localTimeZoneOffsetFromGMTMinute/1 -> Compose String/9

== system NMEA/Decoder/NMEA 0183 Decode  DPT/DecodeMessage ==
  timestamp : Inport
  strID : Inport  Port=2
  depth : Inport  Port=3
  offset : Inport  Port=4
  range : Inport  Port=5
  Enable : EnablePort
  Bus Creator : BusCreator  Inputs=5
  Data Type Conversion : DataTypeConversion  OutDataTypeStr=uint8  SaturateOnIntegerOverflow=off  RndMeth=Floor
  Data Type Conversion{1..4} (4 alike) : DataTypeConversion  OutDataTypeStr=double  SaturateOnIntegerOverflow=off  RndMeth=Floor
  String to ASCII : StringToASCII  OutputVectorSize=2
  DPT : Outport
  wires:
  Data Type Conversion4/1 -> Bus Creator/1  "timestamp"
  Data Type Conversion2/1 -> Bus Creator/4  "offset"
  Data Type Conversion1/1 -> Bus Creator/3  "depth"
  offset/1 -> Data Type Conversion2/1
  depth/1 -> Data Type Conversion1/1
  Data Type Conversion/1 -> Bus Creator/2  "deviceID"
  String to ASCII/1 -> Data Type Conversion/1
  strID/1 -> String to ASCII/1
  timestamp/1 -> Data Type Conversion4/1
  Bus Creator/1 -> DPT/1
  range/1 -> Data Type Conversion3/1
  Data Type Conversion3/1 -> Bus Creator/5  "range"

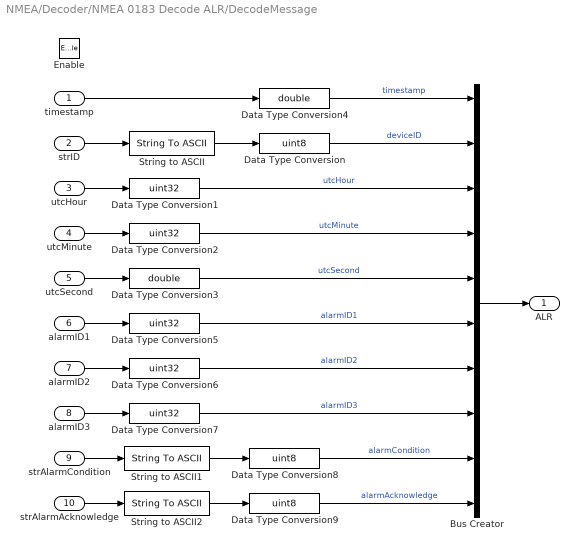
== system NMEA/Decoder/NMEA 0183 Decode ALR/DecodeMessage ==
  timestamp : Inport
  strID : Inport  Port=2
  utcHour : Inport  Port=3
  utcMinute : Inport  Port=4
  utcSecond : Inport  Port=5
  alarmID1 : Inport  Port=6
  alarmID2 : Inport  Port=7
  alarmID3 : Inport  Port=8
  strAlarmCondition : Inport  Port=9
  strAlarmAcknowledge : Inport  Port=10
  Enable : EnablePort
  Bus Creator : BusCreator  Inputs=10
  Data Type Conversion : DataTypeConversion  OutDataTypeStr=uint8  SaturateOnIntegerOverflow=off  RndMeth=Floor
  Data Type Conversion{1..2,5..7} (5 alike) : DataTypeConversion  OutDataTypeStr=uint32  SaturateOnIntegerOverflow=off  RndMeth=Floor
  Data Type Conversion3 : DataTypeConversion  OutDataTypeStr=double  SaturateOnIntegerOverflow=off  RndMeth=Floor
  Data Type Conversion4 : DataTypeConversion  OutDataTypeStr=double  SaturateOnIntegerOverflow=off  RndMeth=Floor
  Data Type Conversion8 : DataTypeConversion  OutDataTypeStr=uint8  SaturateOnIntegerOverflow=off  RndMeth=Floor
  Data Type Conversion9 : DataTypeConversion  OutDataTypeStr=uint8  SaturateOnIntegerOverflow=off  RndMeth=Floor
  String to ASCII : StringToASCII  OutputVectorSize=2
  String to ASCII1 : StringToASCII  OutputVectorSize=1
  String to ASCII2 : StringToASCII  OutputVectorSize=1
  ALR : Outport
  wires:
  Data Type Conversion3/1 -> Bus Creator/5  "utcSecond"
  Data Type Conversion4/1 -> Bus Creator/1  "timestamp"
  Data Type Conversion/1 -> Bus Creator/2  "deviceID"
  String to ASCII/1 -> Data Type Conversion/1
  strID/1 -> String to ASCII/1
  timestamp/1 -> Data Type Conversion4/1
  Bus Creator/1 -> ALR/1
  utcHour/1 -> Data Type Conversion1/1
  utcMinute/1 -> Data Type Conversion2/1
  utcSecond/1 -> Data Type Conversion3/1
  Data Type Conversion1/1 -> Bus Creator/3  "utcHour"
  Data Type Conversion2/1 -> Bus Creator/4  "utcMinute"
  alarmID1/1 -> Data Type Conversion5/1
  alarmID2/1 -> Data Type Conversion6/1
  alarmID3/1 -> Data Type Conversion7/1
  Data Type Conversion5/1 -> Bus Creator/6  "alarmID1"
  Data Type Conversion6/1 -> Bus Creator/7  "alarmID2"
  Data Type Conversion7/1 -> Bus Creator/8  "alarmID3"
  strAlarmCondition/1 -> String to ASCII1/1
  strAlarmAcknowledge/1 -> String to ASCII2/1
  String to ASCII1/1 -> Data Type Conversion8/1
  String to ASCII2/1 -> Data Type Conversion9/1
  Data Type Conversion8/1 -> Bus Creator/9  "alarmCondition"
  Data Type Conversion9/1 -> Bus Creator/10  "alarmAcknowledge"

== system NMEA/Decoder/NMEA 0183 Decode DBT/DecodeMessage ==
  timestamp : Inport
  strID : Inport  Port=2
  depthFeet : Inport  Port=3
  depthMeters : Inport  Port=4
  depthFathoms : Inport  Port=5
  Enable : EnablePort
  Bus Creator : BusCreator  Inputs=5
  Data Type Conversion : DataTypeConversion  OutDataTypeStr=uint8  SaturateOnIntegerOverflow=off  RndMeth=Floor
  Data Type Conversion{1..2,4,11} (4 alike) : DataTypeConversion  OutDataTypeStr=double  SaturateOnIntegerOverflow=off  RndMeth=Floor
  Gain : Gain  Gain=0.304800609601219
  Gain2 : Gain  Gain=1.8288
  String to ASCII : StringToASCII  OutputVectorSize=2
  DBT : Outport
  wires:
  depthFathoms/1 -> Data Type Conversion2/1
  depthMeters/1 -> Data Type Conversion1/1
  depthFeet/1 -> Data Type Conversion11/1
  Data Type Conversion4/1 -> Bus Creator/1  "timestamp"
  Data Type Conversion/1 -> Bus Creator/2  "deviceID"
  String to ASCII/1 -> Data Type Conversion/1
  strID/1 -> String to ASCII/1
  timestamp/1 -> Data Type Conversion4/1
  Bus Creator/1 -> DBT/1
  Data Type Conversion11/1 -> Gain/1
  Gain/1 -> Bus Creator/3  "depth1"
  Data Type Conversion1/1 -> Bus Creator/4  "depth2"
  Data Type Conversion2/1 -> Gain2/1
  Gain2/1 -> Bus Creator/5  "depth3"
